simulink model "Simulink_model"  (R2024b)
settings: Solver=VariableStepAuto  StartTime=0.0  StopTime=20  RelTol=1e-3
values from neighbouring files (symbols this model uses):
  A = [0, 1 ... (first row only)    [Script.m]
  B = [0 ... (first row only)    [Script.m]
  C = [1, 0]    [Script.m]
  D = 0    [Script.m]
  den_filter = [1, 2*delta_filter*omega_filter, omega_filter^2]    [Script.m]
  denH = alpha    [Script.m]
  K_xi = K_z(m+1:end)    [Script.m]
  num_filter = [omega_filter^2, 0]    [Script.m]
undefined symbols (not defined in the file or in its folder): numH
settings Model: Creator=andre  LastModifiedBy=Enrico 2

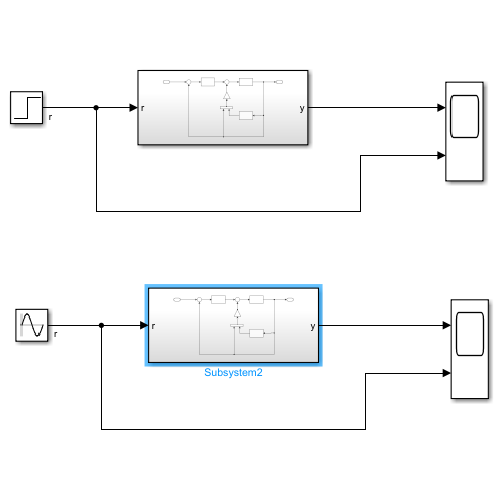
[thumbnail: Simulink's stored preview of the top-level diagram]
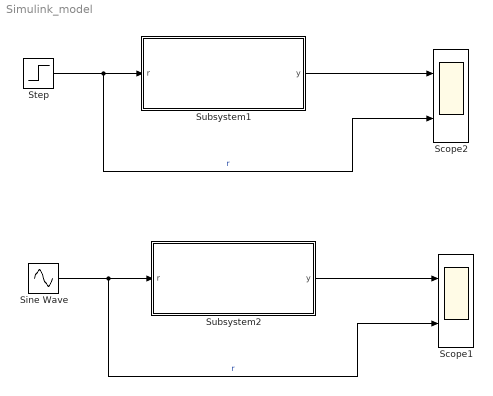
== system Simulink_model ==
  Scope1 : Scope  NumInputPorts=2
  Scope2 : Scope  NumInputPorts=2
  Sine Wave : Sin  Amplitude=40  Frequency=6  SampleTime=0
  Step : Step  After=100  SampleTime=0
  Subsystem1 : Subsystem
  Subsystem2 : Subsystem
  wires:
  Sine Wave/1 -> Subsystem2/1(r), Scope1/2  "r"
  Subsystem1/1(y) -> Scope2/1
  Step/1 -> Subsystem1/1(r), Scope2/2  "r"
  Subsystem2/1(y) -> Scope1/1

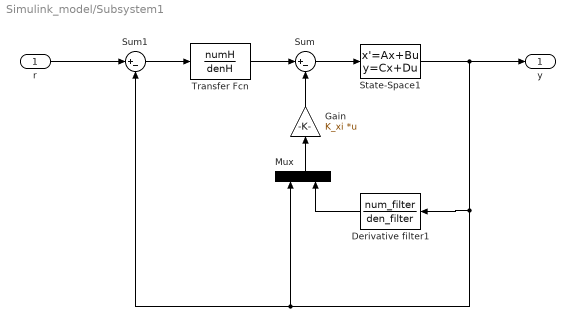
== system Simulink_model/Subsystem1 ==
  r : Inport
  Derivative filter1 : TransferFcn  Numerator=num_filter  Denominator=den_filter
  Gain : Gain  Gain=K_xi  Multiplication=Matrix(K*u)
  Mux : Mux  Inputs=2
  State-Space1 : StateSpace  A=A  B=B  C=C  D=D  InitialCondition=0
  Sum : Sum  Inputs=|+-
  Sum1 : Sum  Inputs=|+-
  Transfer Fcn : TransferFcn  Numerator=numH  Denominator=denH
  y : Outport
  wires:
  Gain/1 -> Sum/2
  Transfer Fcn/1 -> Sum/1
  Mux/1 -> Gain/1
  Sum/1 -> State-Space1/1
  Sum1/1 -> Transfer Fcn/1
  State-Space1/1 -> y/1, Derivative filter1/1, Mux/1, Sum1/2
  r/1 -> Sum1/1
  Derivative filter1/1 -> Mux/2

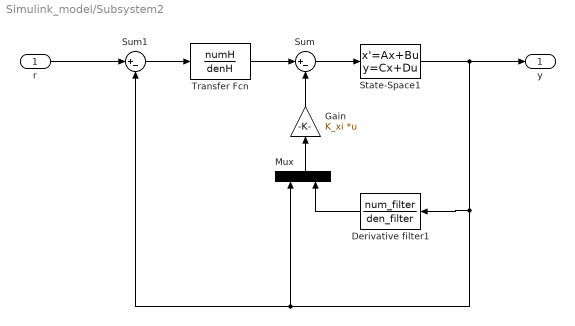
== system Simulink_model/Subsystem2 ==
  r : Inport
  Derivative filter1 : TransferFcn  Numerator=num_filter  Denominator=den_filter
  Gain : Gain  Gain=K_xi  Multiplication=Matrix(K*u)
  Mux : Mux  Inputs=2
  State-Space1 : StateSpace  A=A  B=B  C=C  D=D  InitialCondition=0
  Sum : Sum  Inputs=|+-
  Sum1 : Sum  Inputs=|+-
  Transfer Fcn : TransferFcn  Numerator=numH  Denominator=denH
  y : Outport
  wires:
  Gain/1 -> Sum/2
  Transfer Fcn/1 -> Sum/1
  Mux/1 -> Gain/1
  Sum/1 -> State-Space1/1
  Sum1/1 -> Transfer Fcn/1
  State-Space1/1 -> y/1, Derivative filter1/1, Mux/1, Sum1/2
  r/1 -> Sum1/1
  Derivative filter1/1 -> Mux/2
